simulink model "ysw15_2"  (R2014a)
settings: Solver=ode45  StartTime=0.0  StopTime=10.0  RelTol=1e-3
values from neighbouring files (symbols this model uses):
  A = [0,1,0,-1 ... (first row only)    [ysw15_4.m]    (also in ysw15_5.m)
  B = [0,0,1,0]'    [ysw15_4.m]    (also in ysw15_5.m)
  C = [-8.3859,-4.0703,7.6711,0.1549 ... (first row only)    [ysw15_4.m]    (also in ysw15_5.m = [-66.667,-4.083,0,4.083)
  D = [0,0,0]'    [ysw15_4.m]    (also in ysw15_5.m)
undefined symbols (not defined in the file or in its folder): sigbuilder_block
settings Model: Creator=ii  LastModifiedBy=ii
settings SolverCC: ZeroCrossAlgorithm=Adaptive
settings DebuggingCC: UnderspecifiedInitializationDetection=Classic

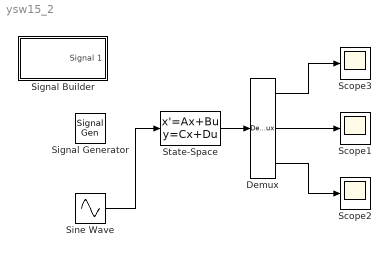
== system ysw15_2 ==
  Demux : Demux  Outputs=3
  Scope1 : Scope
  Scope2 : Scope
  Scope3 : Scope
      settings: SaveName=ScopeData3
  Signal Generator : SignalGenerator  Frequency=10  Units=rad/sec
  Signal Builder : Subsystem  Tag=STV Subsys  LoadFcn=sigbuilder_block('load');  StartFcn=sigbuilder_block('start');  StopFcn=sigbuilder_block('stop');  ClipboardFcn=sigbuilder_block('clipboard');  mask(Sigbuilder block){}
      mask help: Simulink:masks:SigbuilderBlock_MD
      mask init:
      | if ~strcmp(get_param(bdroot(gcbh),'SimulationStatus'),'stopped') tuvar = sigbuilder_block('maskInit'); end
      settings: CopyFcn=sigbuilder_block('copy');  DeleteFcn=sigbuilder_block('delete');  ModelCloseFcn=sigbuilder_block('modelClose');  PreSaveFcn=sigbuilder_block('preSave');  PauseFcn=sigbuilder_block('pause');  ContinueFcn=sigbuilder_block('continue');  NameChangeFcn=sigbuilder_block('namechange');  OpenFcn=sigbuilder_block('open',[188.25 94.5 550.5 393.75 ]);  CloseFcn=sigbuilder_block('close');
      mask Display: plot(0, 0, 100, 100,[2, 2, 32, 32, 2], [68, 8, 8, 68, 68],[32, 2], [38, 38], [32, 19, 2],[53, 60, 44], [32, 17, 17, 2],[16, 16, 31, 31]);txt = getActiveGroup(gcbh);text(2, 100, txt,'verticalAlignment', 'top');
  Sine Wave : Sin  SampleTime=0.01
  State-Space : StateSpace  A=A  B=B  C=C  D=D  X0=0
  wires:
  State-Space/1 -> Demux/1
  Demux/1 -> Scope3/1
  Demux/2 -> Scope1/1
  Demux/3 -> Scope2/1
  Sine Wave/1 -> State-Space/1

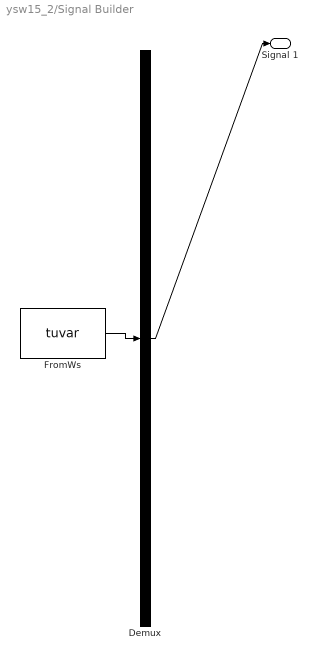
== system ysw15_2/Signal Builder ==
  Demux : Demux  Tag=STV Demux  Outputs=1
  FromWs : FromWorkspace  Tag=STV FromWs  VariableName=tuvar  SampleTime=0
      SigBuilderData=|
      | common.afterFinalStr = 'Extrapolate'
      | common.sampleTime = 0
      | dataSet.timeRange = [0 10]
      | dataSet.name = 'Group 1'
      | sbobj.Groups.Name = 'Group 1'
      | sbobj.Groups.Signals.Name = 'Signal 1'
      | sbobj.Groups.Signals.XData = [0 0.75 0.75 1.45 1.45 2.2 2.2 3.15 3.15 4.05 4.05 4.8 4.8 5.35 5.35 6.05 6.05 6.7 6.7 7.3 7.3 7.8 7.8 8.35 8.35 8.95 8.95 9.65 9.65 10]
      | sbobj.Groups.Signals.YData = [-0.36 -0.355 0.995 0.995 -0.3 -0.295 1.01 1.01 -0.135 -0.135 0.995 0.995 -0.065 -0.065 0.995 0.995 -0.01 -0.01 0.995 0.995 0 0 0.99 0.99 0.015 0.015 0.97 0.97 0.01 0.01]
  Signal 1 : Outport  Tag=STV Outport
  wires:
  FromWs/1 -> Demux/1
  Demux/1 -> Signal 1/1
